simulink model "LQR_Reference_Tracking_Constant_Vx_Cf_Cr_SimContinous"  (R2018a)
settings: Solver=FixedStepAuto  StartTime=0.0  StopTime=t_final  FixedStep=T  RelTol=1e-3
values from neighbouring files (symbols this model uses):
  A = [a11 a12 a13 ... (first row only)    [LQR_Ref_Track_Const_Vx_Cf_Cr_LinMod_3_state.m]    (also in LQR_Ref_Track_Const_Vx_Cf_Cr_LinMod_5_state.m = [0 1 0 0 0; 0 a11 0 a12 0; linearVehicleModel.m; linearVehicleModel2.m; vehicleDeviationModel.m = [0  1  0  0 0)
  B = [b1;b2;b3]    [LQR_Ref_Track_Const_Vx_Cf_Cr_LinMod_3_state.m]    (also in LQR_Ref_Track_Const_Vx_Cf_Cr_LinMod_5_state.m = [0;b1;0;b2;b3]; linearVehicleModel.m; linearVehicleModel2.m; vehicleDeviationModel.m = [0;b1;0;b2;b3])
  K_lqi = lqi(sys,Q,R)    [LQR_Ref_Track_Const_Vx_Cf_Cr_LinMod_3_state.m]    (also in LQR_Ref_Track_Const_Vx_Cf_Cr_LinMod_5_state.m)
  Kc_lqr = Kc(1:3)    [LQR_Ref_Track_Const_Vx_Cf_Cr_LinMod_3_state.m]
  Kic = Kc(4)    [LQR_Ref_Track_Const_Vx_Cf_Cr_LinMod_3_state.m]
undefined symbols (not defined in the file or in its folder): Kc
settings Model: Creator=Shouvik Chakraborty  LastModifiedBy=Shouvik Chakraborty

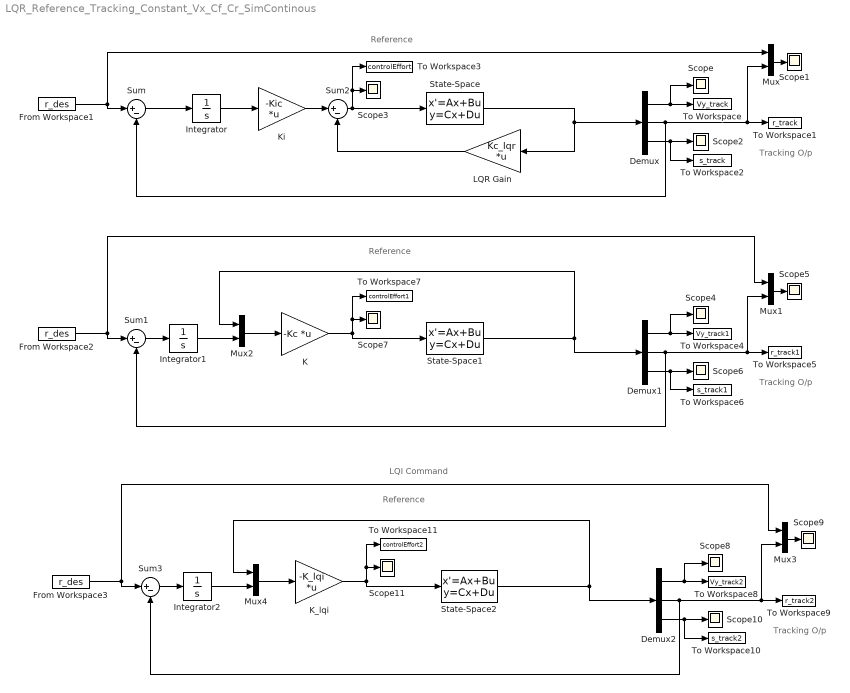
== system LQR_Reference_Tracking_Constant_Vx_Cf_Cr_SimContinous ==
  note: LQI Command
  note: Reference
  note: Tracking O/p
  note: Reference
  note: Tracking O/p
  note: Tracking O/p
  note: Reference
  Demux : Demux  Outputs=3
  Demux1 : Demux  Outputs=3
  Demux2 : Demux  Outputs=3
  From Workspace1 : FromWorkspace  VariableName=r_des  SampleTime=0
  From Workspace2 : FromWorkspace  VariableName=r_des  SampleTime=0
  From Workspace3 : FromWorkspace  VariableName=r_des  SampleTime=0
  Integrator : Integrator
  Integrator1 : Integrator
  Integrator2 : Integrator
  K : Gain  Gain=-Kc  Multiplication=Matrix(K*u)
  K_lqi : Gain  Gain=-K_lqi  Multiplication=Matrix(K*u)
  Ki : Gain  Gain=-Kic  Multiplication=Matrix(K*u)
  LQR Gain : Gain  Gain=Kc_lqr  Multiplication=Matrix(K*u)
  Mux{,1..4} (5 alike) : Mux  Inputs=2
  Scope{,1..11} (12 alike) : Scope
  State-Space : StateSpace  A=A  B=B  C=eye(3,3)  D=[0; 0; 0]  InitialCondition=0
  State-Space1 : StateSpace  A=A  B=B  C=eye(3,3)  D=[0; 0; 0]  InitialCondition=0
  State-Space2 : StateSpace  A=A  B=B  C=eye(3,3)  D=[0; 0; 0]  InitialCondition=0
  Sum{,1..3} (4 alike) : Sum  Inputs=|+-
  To Workspace : ToWorkspace  VariableName=Vy_track  SampleTime=-1
  To Workspace1 : ToWorkspace  VariableName=r_track  SampleTime=-1
  To Workspace10 : ToWorkspace  VariableName=s_track2  SampleTime=-1
  To Workspace11 : ToWorkspace  VariableName=controlEffort2  SampleTime=-1
  To Workspace2 : ToWorkspace  VariableName=s_track  SampleTime=-1
  To Workspace3 : ToWorkspace  VariableName=controlEffort  SampleTime=-1
  To Workspace4 : ToWorkspace  VariableName=Vy_track1  SampleTime=-1
  To Workspace5 : ToWorkspace  VariableName=r_track1  SampleTime=-1
  To Workspace6 : ToWorkspace  VariableName=s_track1  SampleTime=-1
  To Workspace7 : ToWorkspace  VariableName=controlEffort1  SampleTime=-1
  To Workspace8 : ToWorkspace  VariableName=Vy_track2  SampleTime=-1
  To Workspace9 : ToWorkspace  VariableName=r_track2  SampleTime=-1
  wires:
  Demux/1 -> Scope/1, To Workspace/1
  Sum/1 -> Integrator/1
  Integrator/1 -> Ki/1
  Sum2/1 -> State-Space/1, To Workspace3/1, Scope3/1
  State-Space/1 -> Demux/1, LQR Gain/1
  LQR Gain/1 -> Sum2/2
  From Workspace1/1 -> Sum/1, Mux/1
  Ki/1 -> Sum2/1
  Demux/2 -> Sum/2, Mux/2, To Workspace1/1
  Demux/3 -> To Workspace2/1, Scope2/1
  Mux/1 -> Scope1/1
  Mux1/1 -> Scope5/1
  Demux1/1 -> Scope4/1, To Workspace4/1
  Demux1/2 -> Sum1/2, Mux1/2, To Workspace5/1
  Demux1/3 -> To Workspace6/1, Scope6/1
  State-Space1/1 -> Demux1/1, Mux2/1
  From Workspace2/1 -> Sum1/1, Mux1/1
  K/1 -> State-Space1/1, To Workspace7/1, Scope7/1
  Sum1/1 -> Integrator1/1
  Integrator1/1 -> Mux2/2
  Mux2/1 -> K/1
  Mux4/1 -> K_lqi/1
  State-Space2/1 -> Demux2/1, Mux4/1
  Sum3/1 -> Integrator2/1
  From Workspace3/1 -> Sum3/1, Mux3/1
  Demux2/3 -> To Workspace10/1, Scope10/1
  K_lqi/1 -> State-Space2/1, To Workspace11/1, Scope11/1
  Demux2/1 -> Scope8/1, To Workspace8/1
  Mux3/1 -> Scope9/1
  Demux2/2 -> Sum3/2, Mux3/2, To Workspace9/1
  Integrator2/1 -> Mux4/2
